simulink model "Scheme_FDr21a"  (R2021b)
settings: Solver=VariableStepAuto  StartTime=0.0  StopTime=2  RelTol=1e-3
values from neighbouring files (symbols this model uses):
  g = 9.81    [init.m]
  L = 2    [init.m]
  M = 5    [init.m]
  m = 1    [init.m]
settings Model: Creator=fabri  LastModifiedBy=brizio
settings DebuggingCC: UnconnectedInputMsg=none  UnconnectedOutputMsg=none  UnconnectedLineMsg=none
settings ModelReferenceCC: EnableRefExpFcnMdlSchedulingChecks=off
settings RTWCC: DLArmComputeVersion=20.02.1

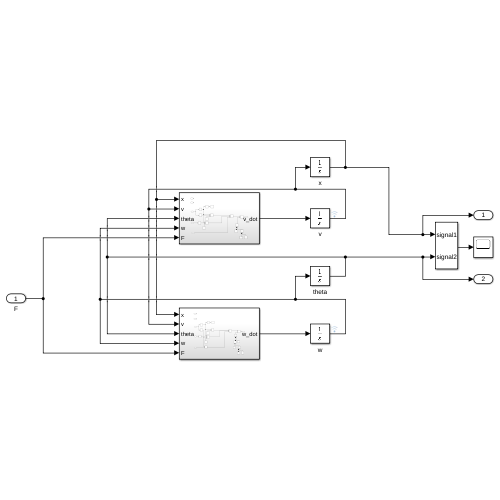
[thumbnail: Simulink's stored preview of the top-level diagram]
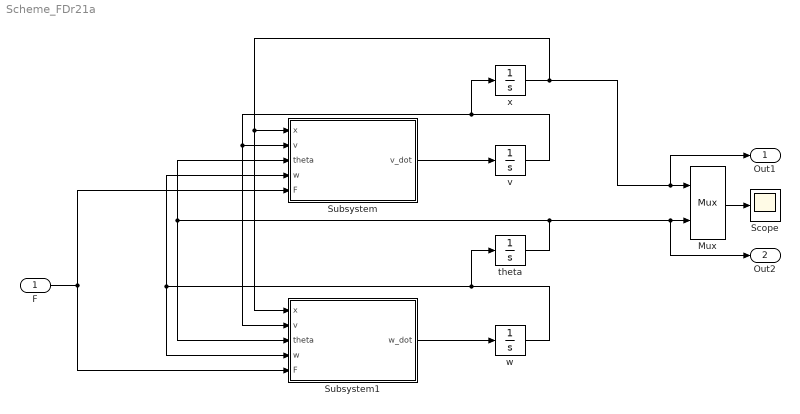
== system Scheme_FDr21a ==
  F : Inport
  Mux : Mux  Inputs=2
      settings: DisplayOption=signals
  Scope : Scope
  Subsystem : Subsystem
  Subsystem1 : Subsystem
  theta : Integrator  InitialCondition=3.04
  v : Integrator
  w : Integrator
  x : Integrator
  Out1 : Outport
  Out2 : Outport  Port=2
  wires:
  theta/1 -> Subsystem/3(theta), Subsystem1/3(theta), Out2/1, Mux/2
  x/1 -> Out1/1, Mux/1, Subsystem1/1(x), Subsystem/1(x)
  F/1 -> Subsystem/5(F), Subsystem1/5(F)
  Mux/1 -> Scope/1
  Subsystem/1(v_dot) -> v/1
  Subsystem1/1(w_dot) -> w/1
  w/1 -> Subsystem1/4(w), Subsystem/4(w), theta/1
  v/1 -> Subsystem/2(v), Subsystem1/2(v), x/1

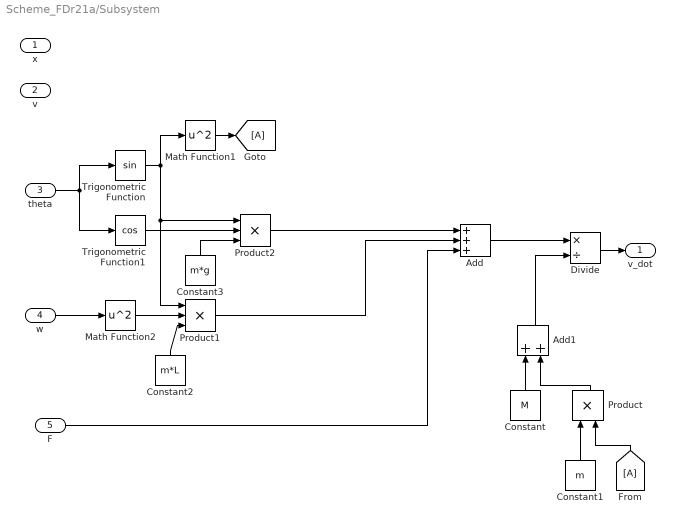
== system Scheme_FDr21a/Subsystem ==
  x : Inport
  v : Inport  Port=2
  theta : Inport  Port=3
  w : Inport  Port=4
  F : Inport  Port=5
  Add : Sum  Inputs=+++
  Add1 : Sum
  Constant : Constant  Value=M
  Constant1 : Constant  Value=m
  Constant2 : Constant  Value=m*L
  Constant3 : Constant  Value=m*g
  Divide : Product  Inputs=*/
  Math Function1 : Math  Operator=square  SaturateOnIntegerOverflow=on
  Math Function2 : Math  Operator=square  SaturateOnIntegerOverflow=on
  Product : Product
  Product1 : Product  Inputs=3
  Product2 : Product  Inputs=3
  Trigonometric Function : Trigonometry
  Trigonometric Function1 : Trigonometry  Operator=cos
  v_dot : Outport
  wires:
  Divide/1 -> v_dot/1
  Add1/1 -> Divide/2
  Constant/1 -> Add1/1
  Product/1 -> Add1/2
  theta/1 -> Trigonometric Function1/1, Trigonometric Function/1
  Trigonometric Function/1 -> Product1/1, Product2/1, Math Function1/1
  w/1 -> Math Function2/1
  Math Function1/1 -> [A]
  [A] -> Product/2
  Constant1/1 -> Product/1
  Math Function2/1 -> Product1/2
  Constant2/1 -> Product1/3
  Add/1 -> Divide/1
  Trigonometric Function1/1 -> Product2/2
  Constant3/1 -> Product2/3
  Product1/1 -> Add/2
  Product2/1 -> Add/1
  F/1 -> Add/3

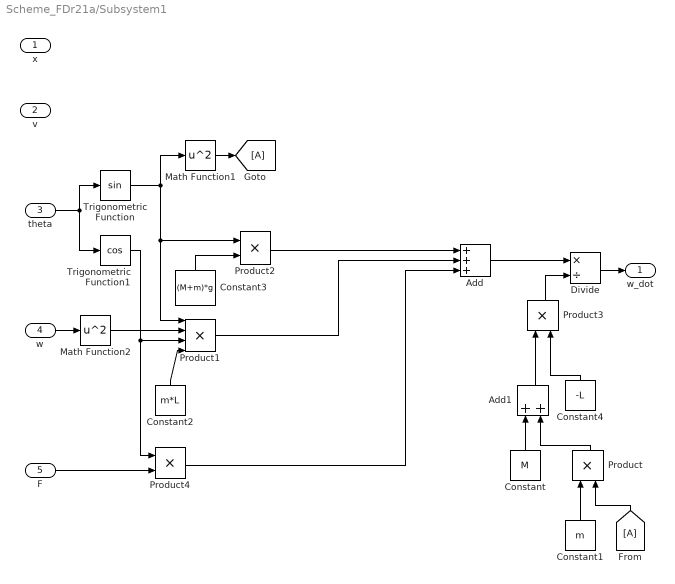
== system Scheme_FDr21a/Subsystem1 ==
  x : Inport
  v : Inport  Port=2
  theta : Inport  Port=3
  w : Inport  Port=4
  F : Inport  Port=5
  Add : Sum  Inputs=+++
  Add1 : Sum
  Constant : Constant  Value=M
  Constant1 : Constant  Value=m
  Constant2 : Constant  Value=m*L
  Constant3 : Constant  Value=(M+m)*g
  Constant4 : Constant  Value=-L
  Divide : Product  Inputs=*/
  Math Function1 : Math  Operator=square  SaturateOnIntegerOverflow=on
  Math Function2 : Math  Operator=square  SaturateOnIntegerOverflow=on
  Product{,2..4} (4 alike) : Product
  Product1 : Product  Inputs=4
  Trigonometric Function : Trigonometry
  Trigonometric Function1 : Trigonometry  Operator=cos
  w_dot : Outport
  wires:
  Divide/1 -> w_dot/1
  Constant/1 -> Add1/1
  Product/1 -> Add1/2
  theta/1 -> Trigonometric Function1/1, Trigonometric Function/1
  Trigonometric Function/1 -> Product1/1, Product2/1, Math Function1/1
  w/1 -> Math Function2/1
  Math Function1/1 -> [A]
  [A] -> Product/2
  Constant1/1 -> Product/1
  Math Function2/1 -> Product1/2
  Add/1 -> Divide/1
  Trigonometric Function1/1 -> Product1/3, Product4/1
  Constant3/1 -> Product2/2
  Product1/1 -> Add/2
  Product2/1 -> Add/1
  Add1/1 -> Product3/1
  Product3/1 -> Divide/2
  Constant4/1 -> Product3/2
  F/1 -> Product4/2
  Product4/1 -> Add/3
  Constant2/1 -> Product1/4
